simulink model "PID"  (R2023a)
settings: Solver=VariableStepAuto  StartTime=0.0  StopTime=30  RelTol=1e-3
settings Model: Creator=c  LastModifiedBy=c

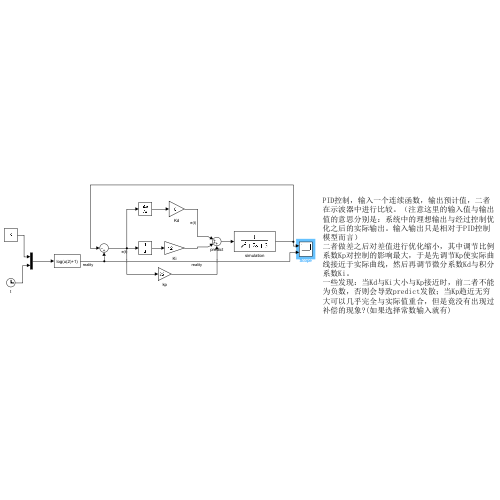
[thumbnail: Simulink's stored preview of the top-level diagram]
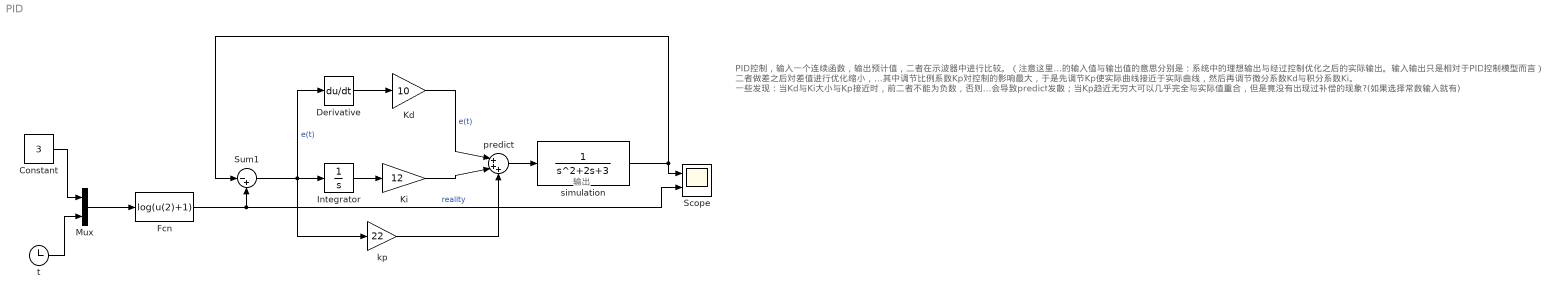
== system PID ==
  note: 输出
  note: PID控制，输入一个连续函数，输出预计值，二者在示波器中进行比较。（注意这里的输入值与输出值的意思分别是：系统中的理想输出与经过控制优化之后的实际输出。输入输出只是相对于PID控制模型而言）
      | 二者做差之后对差值进行优化缩小，其中调节比例系数Kp对控制的影响最大，于是先调节Kp使实际曲线接近于实际曲线，然后再调节微分系数Kd与积分系数Ki。
      | 一些发现：当Kd与Ki大小与Kp接近时，前二者不能为负数，否则会导致predict发散；当Kp趋近无穷大可以几乎完全与实际值重合，但是竟没有出现过补偿的现象?(如果选择常数输入就有)
  Constant : Constant  Value=3
  Derivative : Derivative
  Fcn : Fcn  Expr=log(u(2)+1)
  Integrator : Integrator
  Kd : Gain  Gain=10
  Ki : Gain  Gain=12
  Mux : Mux  Inputs=2
  Scope : Scope  NumInputPorts=2
  Sum1 : Sum  Inputs=|-+
  kp : Gain  Gain=22
  predict : Sum  Inputs=|+++
  simulation : TransferFcn  Denominator=[1 2 3]
  t : Clock
  wires:
  predict/1 -> simulation/1
  Kd/1 -> predict/1  "e(t)"
  Ki/1 -> predict/2
  Integrator/1 -> Ki/1
  kp/1 -> predict/3
  Sum1/1 -> Derivative/1, kp/1, Integrator/1  "e(t)"
  Derivative/1 -> Kd/1
  Fcn/1 -> Sum1/2, Scope/2  "reality"
  Constant/1 -> Mux/1
  t/1 -> Mux/2
  Mux/1 -> Fcn/1
  simulation/1 -> Sum1/1, Scope/1
